simulink model "linearisedmodel"  (R2020b)
settings: Solver=VariableStepAuto  StartTime=0.0  StopTime=10.0  RelTol=1e-3
values from neighbouring files (symbols this model uses):
  b = 2.8956    [myworkspace.mat]    (also in param_uav_updated.m)
  eve = 134.75    [myworkspace.mat]    (also in param_uav_updated.m = (rho.*Va^2.*S_wing/2))
  g = 9.80665    [dyn_nlin.m]    (also in myworkspace.mat = 9.81; param_uav_updated.m; uav_eom_linear_param.m)
  P =     [myworkspace.mat]    (also in param_uav_updated.m = structure of all parameters for the Aerosonde UAV vehicle de; uav_eom_linear_param.m = param_uav_updated2(alpha))
  Va = sqrt(u^2+v^2+w^2)    [dyn_nlin.m]    (also in myworkspace.mat = 20; param_uav_updated.m = 20)
libraries: shared6dof x1, simulink x1
settings Model: Creator=Obian  LastModifiedBy=Obian

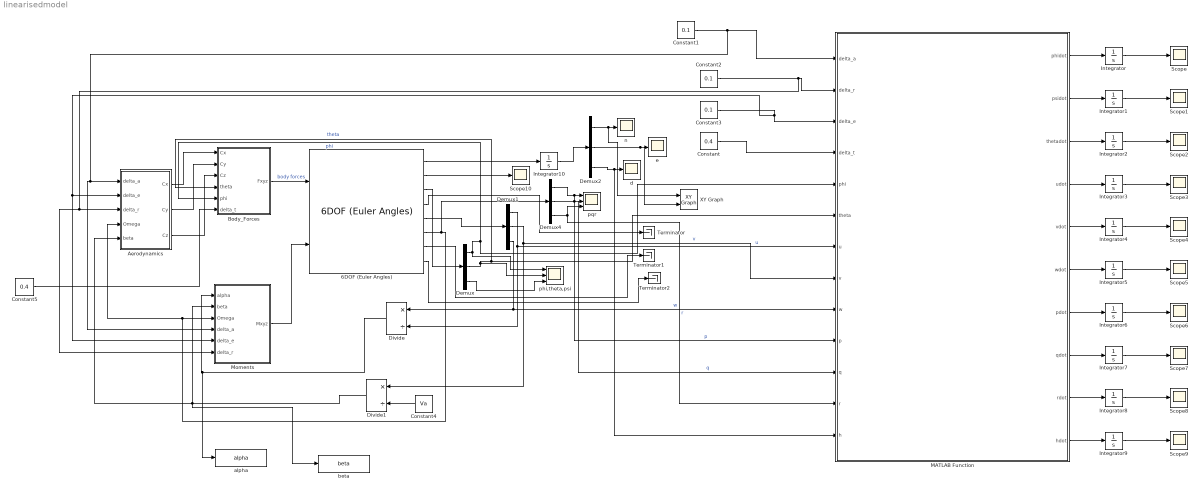
== system linearisedmodel ==
  6DOF (Euler Angles) : shared6dof/6DOF (Euler Angles)  units=Metric (MKS)  mtype=Fixed  rep=Euler Angles  xme_0=[0 0 100]  Vm_0=[20 0 0]  eul_0=[0 0 0]  pm_0=[0 0 0]  mass_0=P.mass  mass_e=0.5  mass_f=2.0  inertia=[P.Jx 0 0; 0 P.Jy 0; 0 0 P.Jz]  inertia_e=eye(3)  inertia_f=2*eye(3)  k_quat=1.0  vre_flag=on  abi_flag=off  aMode=0  xme_statename=''  Vm_statename=''  eul_statename=''  quat_statename=''  pm_statename=''  mass_statename=''
      settings: SourceProductBaseCode=AE,PW,MT,UV,VE,VP
  Aerodynamics : Subsystem
  Body_Forces : Subsystem
  Constant : Constant  Value=0.4
  Constant1 : Constant  Value=0.1
  Constant2 : Constant  Value=0.1
  Constant3 : Constant  Value=0.1
  Constant4 : Constant  Value=Va
  Constant5 : Constant  Value=0.4
  Demux{,1..2,4} (4 alike) : Demux  Outputs=3
  Divide : Product  Inputs=*/
  Divide1 : Product  Inputs=*/
  Integrator{,1..10} (11 alike) : Integrator
  MATLAB Function : MATLAB Function  TreatAsAtomicUnit=on
  Moments : Subsystem
  Scope{,1..10} (11 alike) : Scope
  Terminator : Terminator
  Terminator1 : Terminator
  Terminator2 : Terminator
  XY Graph : simulink/Sinks/XY Graph  xmin=-800  xmax=0  ymin=0  ymax=2500  st=0.01
  alpha : ToWorkspace  VariableName=alpha  SaveFormat=Timeseries  SampleTime=-1
  beta : ToWorkspace  VariableName=beta  SaveFormat=Timeseries  SampleTime=-1
  d : Scope
  e : Scope
  n : Scope
  phi,theta,psi : Scope  NumInputPorts=3
  pqr : Scope  NumInputPorts=3
  wires:
  Constant/1 -> MATLAB Function/4(delta_t)
  Integrator9/1 -> Scope9/1
  Integrator8/1 -> Scope8/1
  Integrator/1 -> Scope/1
  Integrator1/1 -> Scope1/1
  Integrator2/1 -> Scope2/1
  Integrator3/1 -> Scope3/1
  Integrator4/1 -> Scope4/1
  Integrator5/1 -> Scope5/1
  Integrator6/1 -> Scope6/1
  Integrator7/1 -> Scope7/1
  MATLAB Function/1(phidot) -> Integrator/1
  MATLAB Function/2(psidot) -> Integrator1/1
  MATLAB Function/3(thetadot) -> Integrator2/1
  MATLAB Function/4(udot) -> Integrator3/1
  MATLAB Function/5(vdot) -> Integrator4/1
  MATLAB Function/6(wdot) -> Integrator5/1
  MATLAB Function/7(pdot) -> Integrator6/1
  MATLAB Function/8(qdot) -> Integrator7/1
  MATLAB Function/9(rdot) -> Integrator8/1
  MATLAB Function/10(hdot) -> Integrator9/1
  Constant1/1 -> Moments/4(delta_a), Aerodynamics/1(delta_a), MATLAB Function/1(delta_a)
  6DOF (Euler Angles)/8 -> Terminator2/1
  6DOF (Euler Angles)/5 -> Demux1/1
  6DOF (Euler Angles)/4 -> Terminator/1
  6DOF (Euler Angles)/7 -> Terminator1/1
  6DOF (Euler Angles)/2 -> Scope10/1
  Demux4/1 -> MATLAB Function/10(p), pqr/1  "p"
  Demux4/3 -> MATLAB Function/12(r), pqr/3  "r"
  Divide1/1 -> beta/1, Moments/2(beta), Aerodynamics/5(beta)
  Constant3/1 -> Moments/5(delta_e), Aerodynamics/2(delta_e), MATLAB Function/3(delta_e)
  Integrator10/1 -> Demux2/1
  Constant5/1 -> Body_Forces/6(delta_t)
  Demux2/1 -> XY Graph/1, n/1
  6DOF (Euler Angles)/1 -> Integrator10/1
  Demux2/2 -> XY Graph/2, e/1
  Constant4/1 -> Divide1/2
  Demux2/3 -> MATLAB Function/13(h), d/1
  Divide/1 -> alpha/1, Moments/1(alpha)
  Demux/3 -> phi,theta,psi/3
  Demux1/2 -> Divide1/1, MATLAB Function/8(v)  "v"
  Demux/2 -> Body_Forces/4(theta), MATLAB Function/6(theta), phi,theta,psi/2  "theta"
  Demux/1 -> Body_Forces/5(phi), MATLAB Function/5(phi), phi,theta,psi/1  "phi"
  6DOF (Euler Angles)/3 -> Demux/1
  6DOF (Euler Angles)/6 -> Demux4/1, Aerodynamics/4(Omega), Moments/3(Omega)
  Aerodynamics/1(Cx) -> Body_Forces/1(Cx)
  Moments/1(Mxyz) -> 6DOF (Euler Angles)/2
  Body_Forces/1(Fxyz) -> 6DOF (Euler Angles)/1  "body forces"
  Demux4/2 -> MATLAB Function/11(q), pqr/2  "q"
  Aerodynamics/3(Cz) -> Body_Forces/3(Cz)
  Demux1/1 -> MATLAB Function/7(u), Divide/2  "u"
  Aerodynamics/2(Cy) -> Body_Forces/2(Cy)
  Demux1/3 -> MATLAB Function/9(w), Divide/1  "w"
  Constant2/1 -> Moments/6(delta_r), Aerodynamics/3(delta_r), MATLAB Function/2(delta_r)

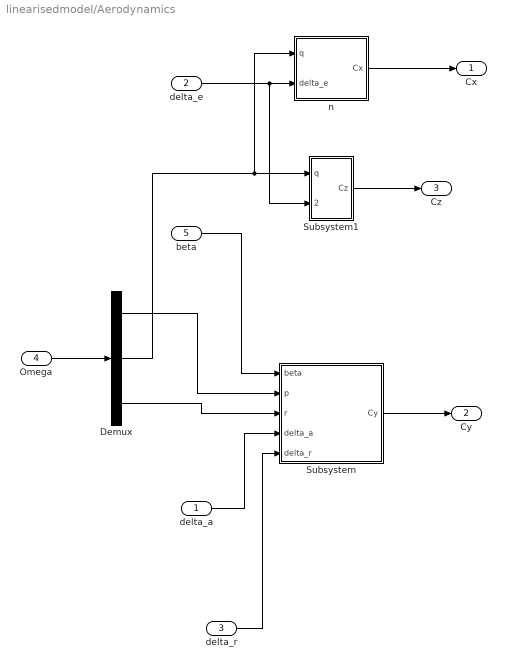
== system linearisedmodel/Aerodynamics ==
  delta_a : Inport
  delta_e : Inport  Port=2
  delta_r : Inport  Port=3
  Omega : Inport  Port=4
  beta : Inport  Port=5
  Demux : Demux  Outputs=3
  Subsystem : Subsystem
  Subsystem1 : Subsystem
  n : Subsystem
  Cx : Outport
  Cy : Outport  Port=2
  Cz : Outport  Port=3
  wires:
  Demux/2 -> n/1(q), Subsystem1/1(q)
  beta/1 -> Subsystem/1(beta)
  delta_a/1 -> Subsystem/4(delta_a)
  delta_e/1 -> Subsystem1/2(delta_e), n/2(delta_e)
  delta_r/1 -> Subsystem/5(delta_r)
  n/1(Cx) -> Cx/1
  Subsystem1/1(Cz) -> Cz/1
  Subsystem/1(Cy) -> Cy/1
  Demux/1 -> Subsystem/2(p)
  Demux/3 -> Subsystem/3(r)
  Omega/1 -> Demux/1

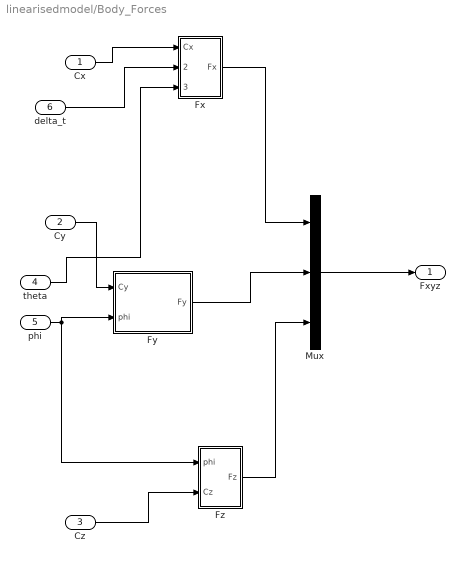
== system linearisedmodel/Body_Forces ==
  Cx : Inport
  Cy : Inport  Port=2
  Cz : Inport  Port=3
  theta : Inport  Port=4
  phi : Inport  Port=5
  delta_t : Inport  Port=6
  Fx : Subsystem
  Fy : Subsystem
  Fz : Subsystem
  Mux : Mux  Inputs=3
  Fxyz : Outport
  wires:
  Cx/1 -> Fx/1(Cx)
  Fx/1(Fx) -> Mux/1
  phi/1 -> Fz/1(phi), Fy/2(phi)
  theta/1 -> Fx/3(theta)
  Cy/1 -> Fy/1(Cy)
  Fy/1(Fy) -> Mux/2
  Fz/1(Fz) -> Mux/3
  Mux/1 -> Fxyz/1
  Cz/1 -> Fz/2(Cz)
  delta_t/1 -> Fx/2(delta_t)

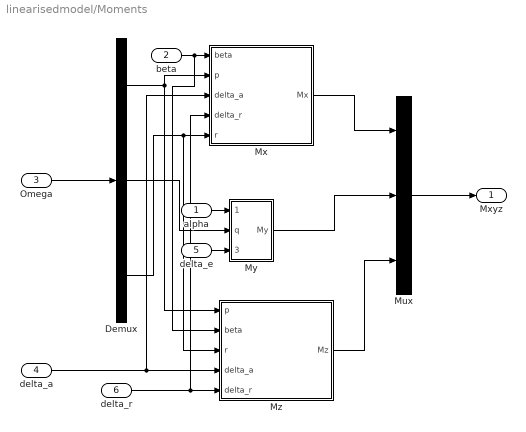
== system linearisedmodel/Moments ==
  alpha : Inport
  beta : Inport  Port=2
  Omega : Inport  Port=3
  delta_a : Inport  Port=4
  delta_e : Inport  Port=5
  delta_r : Inport  Port=6
  Demux : Demux  Outputs=3
  Mux : Mux  Inputs=3
  Mx : Subsystem
  My : Subsystem
  Mz : Subsystem
  Mxyz : Outport
  wires:
  delta_a/1 -> Mx/3(delta_a), Mz/4(delta_a)
  Mz/1(Mz) -> Mux/3
  Demux/2 -> My/2(q)
  Demux/3 -> Mz/3(r), Mx/5(r)
  Demux/1 -> Mz/1(p), Mx/2(p)
  delta_e/1 -> My/3(delta_e)
  delta_r/1 -> Mx/4(delta_r), Mz/5(delta_r)
  alpha/1 -> My/1(alpha)
  Mx/1(Mx) -> Mux/1
  Omega/1 -> Demux/1
  My/1(My) -> Mux/2
  Mux/1 -> Mxyz/1
  beta/1 -> Mz/2(beta), Mx/1(beta)

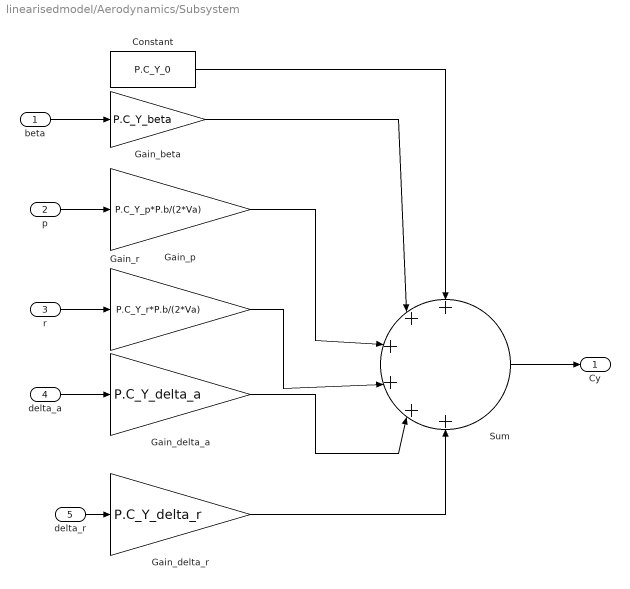
== system linearisedmodel/Aerodynamics/Subsystem ==
  beta : Inport
  p : Inport  Port=2
  r : Inport  Port=3
  delta_a : Inport  Port=4
  delta_r : Inport  Port=5
  Constant : Constant  Value=P.C_Y_0
  Gain_beta : Gain  Gain=P.C_Y_beta
  Gain_delta_a : Gain  Gain=P.C_Y_delta_a
  Gain_delta_r : Gain  Gain=P.C_Y_delta_r
  Gain_p : Gain  Gain=P.C_Y_p*P.b/(2*Va)
  Gain_r : Gain  Gain=P.C_Y_r*P.b/(2*Va)
  Sum : Sum  Inputs=++++++
  Cy : Outport
  wires:
  p/1 -> Gain_p/1
  Gain_r/1 -> Sum/4
  Gain_beta/1 -> Sum/2
  Gain_p/1 -> Sum/3
  delta_a/1 -> Gain_delta_a/1
  beta/1 -> Gain_beta/1
  Gain_delta_r/1 -> Sum/6
  Sum/1 -> Cy/1
  r/1 -> Gain_r/1
  Constant/1 -> Sum/1
  Gain_delta_a/1 -> Sum/5
  delta_r/1 -> Gain_delta_r/1

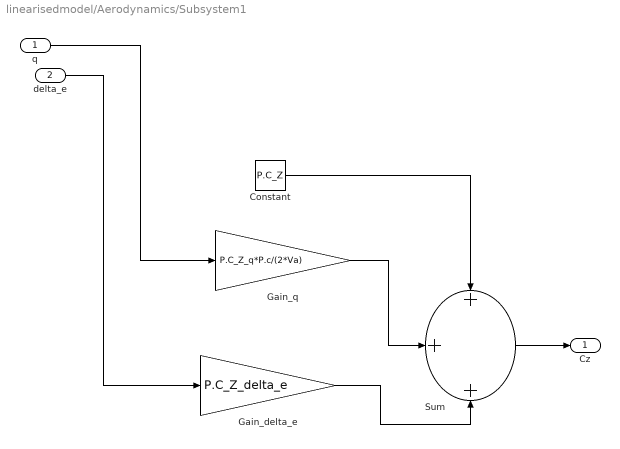
== system linearisedmodel/Aerodynamics/Subsystem1 ==
  q : Inport
  delta_e : Inport  Port=2
  Constant : Constant  Value=P.C_Z
  Gain_delta_e : Gain  Gain=P.C_Z_delta_e
  Gain_q : Gain  Gain=P.C_Z_q*P.c/(2*Va)
  Sum : Sum  Inputs=+++
  Cz : Outport
  wires:
  Sum/1 -> Cz/1
  Gain_q/1 -> Sum/2
  Gain_delta_e/1 -> Sum/3
  Constant/1 -> Sum/1
  delta_e/1 -> Gain_delta_e/1
  q/1 -> Gain_q/1

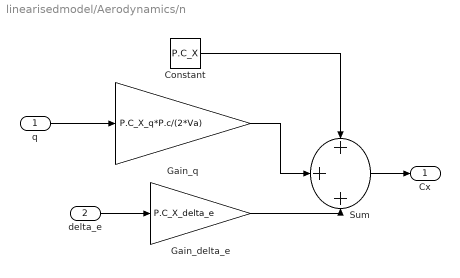
== system linearisedmodel/Aerodynamics/n ==
  q : Inport
  delta_e : Inport  Port=2
  Constant : Constant  Value=P.C_X
  Gain_delta_e : Gain  Gain=P.C_X_delta_e
  Gain_q : Gain  Gain=P.C_X_q*P.c/(2*Va)
  Sum : Sum  Inputs=+++
  Cx : Outport
  wires:
  Constant/1 -> Sum/1
  Gain_delta_e/1 -> Sum/3
  q/1 -> Gain_q/1
  Sum/1 -> Cx/1
  Gain_q/1 -> Sum/2
  delta_e/1 -> Gain_delta_e/1

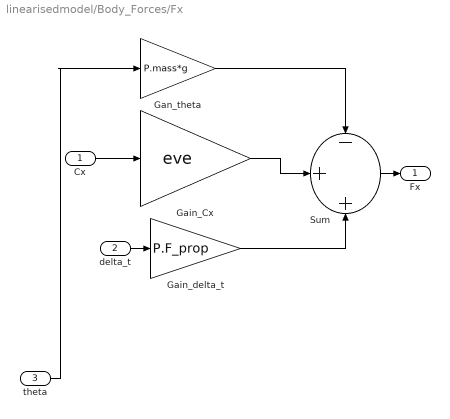
== system linearisedmodel/Body_Forces/Fx ==
  Cx : Inport
  delta_t : Inport  Port=2
  theta : Inport  Port=3
  Gain_Cx : Gain  Gain=eve
  Gain_delta_t : Gain  Gain=P.F_prop
  Gan_theta : Gain  Gain=P.mass*g
  Sum : Sum  Inputs=-++
  Fx : Outport
  wires:
  Gan_theta/1 -> Sum/1
  Gain_Cx/1 -> Sum/2
  Gain_delta_t/1 -> Sum/3
  Cx/1 -> Gain_Cx/1
  delta_t/1 -> Gain_delta_t/1
  Sum/1 -> Fx/1
  theta/1 -> Gan_theta/1

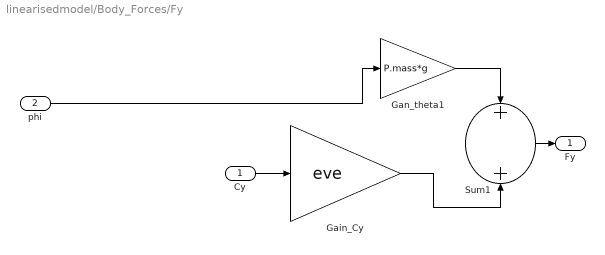
== system linearisedmodel/Body_Forces/Fy ==
  Cy : Inport
  phi : Inport  Port=2
  Gain_Cy : Gain  Gain=eve
  Gan_theta1 : Gain  Gain=P.mass*g
  Sum1 : Sum
  Fy : Outport
  wires:
  Gan_theta1/1 -> Sum1/1
  Sum1/1 -> Fy/1
  Cy/1 -> Gain_Cy/1
  Gain_Cy/1 -> Sum1/2
  phi/1 -> Gan_theta1/1

== system linearisedmodel/Body_Forces/Fz ==
  phi : Inport
  Cz : Inport  Port=2
  Gain_Cz : Gain  Gain=eve
  Gan_theta1 : Gain  Gain=P.mass*g
  Sum1 : Sum
  Fz : Outport
  wires:
  Gain_Cz/1 -> Sum1/2
  Cz/1 -> Gain_Cz/1
  Sum1/1 -> Fz/1
  Gan_theta1/1 -> Sum1/1
  phi/1 -> Gan_theta1/1

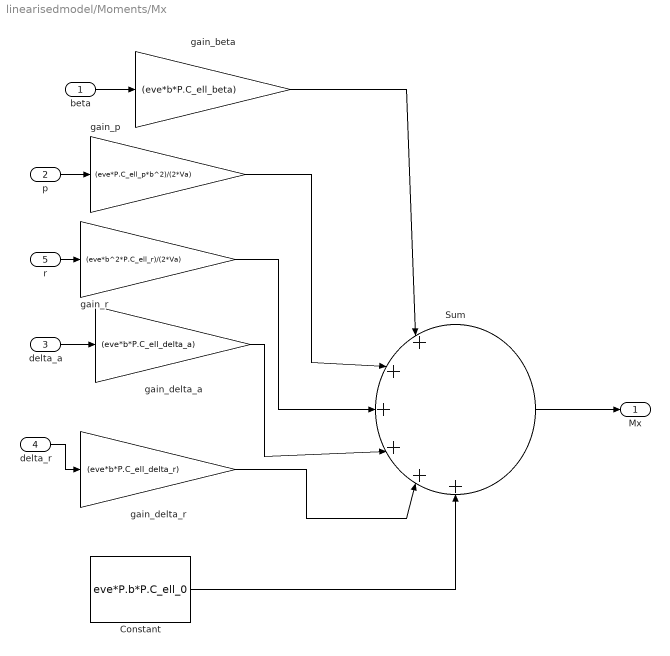
== system linearisedmodel/Moments/Mx ==
  beta : Inport
  p : Inport  Port=2
  delta_a : Inport  Port=3
  delta_r : Inport  Port=4
  r : Inport  Port=5
  Constant : Constant  Value=eve*P.b*P.C_ell_0
  Sum : Sum  Inputs=|++++++
  gain_beta : Gain  Gain=(eve*b*P.C_ell_beta)
  gain_delta_a : Gain  Gain=(eve*b*P.C_ell_delta_a)
  gain_delta_r : Gain  Gain=(eve*b*P.C_ell_delta_r)
  gain_p : Gain  Gain=(eve*P.C_ell_p*b^2)/(2*Va)
  gain_r : Gain  Gain=(eve*b^2*P.C_ell_r)/(2*Va)
  Mx : Outport
  wires:
  gain_beta/1 -> Sum/1
  delta_r/1 -> gain_delta_r/1
  p/1 -> gain_p/1
  r/1 -> gain_r/1
  gain_p/1 -> Sum/2
  delta_a/1 -> gain_delta_a/1
  gain_r/1 -> Sum/3
  beta/1 -> gain_beta/1
  gain_delta_r/1 -> Sum/5
  Sum/1 -> Mx/1
  Constant/1 -> Sum/6
  gain_delta_a/1 -> Sum/4

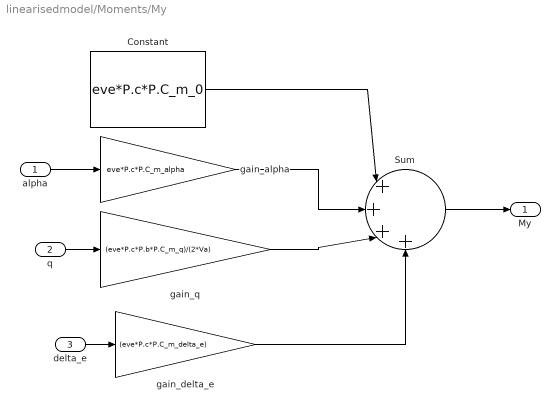
== system linearisedmodel/Moments/My ==
  alpha : Inport
  q : Inport  Port=2
  delta_e : Inport  Port=3
  Constant : Constant  Value=eve*P.c*P.C_m_0
  Sum : Sum  Inputs=|++++
  gain_alpha : Gain  Gain=eve*P.c*P.C_m_alpha
  gain_delta_e : Gain  Gain=(eve*P.c*P.C_m_delta_e)
  gain_q : Gain  Gain=(eve*P.c*P.b*P.C_m_q)/(2*Va)
  My : Outport
  wires:
  Sum/1 -> My/1
  gain_delta_e/1 -> Sum/4
  gain_q/1 -> Sum/3
  q/1 -> gain_q/1
  delta_e/1 -> gain_delta_e/1
  gain_alpha/1 -> Sum/2
  Constant/1 -> Sum/1
  alpha/1 -> gain_alpha/1

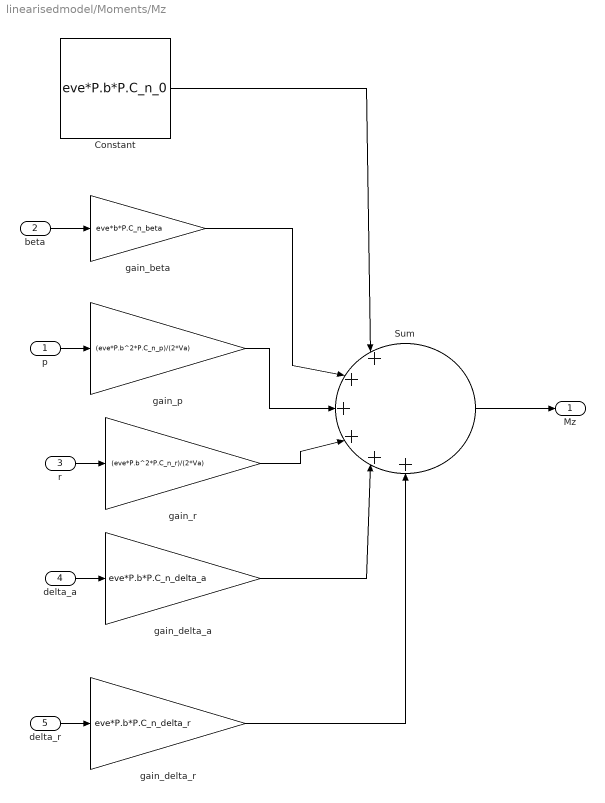
== system linearisedmodel/Moments/Mz ==
  p : Inport
  beta : Inport  Port=2
  r : Inport  Port=3
  delta_a : Inport  Port=4
  delta_r : Inport  Port=5
  Constant : Constant  Value=eve*P.b*P.C_n_0
  Sum : Sum  Inputs=|++++++
  gain_beta : Gain  Gain=eve*b*P.C_n_beta
  gain_delta_a : Gain  Gain=eve*P.b*P.C_n_delta_a
  gain_delta_r : Gain  Gain=eve*P.b*P.C_n_delta_r
  gain_p : Gain  Gain=(eve*P.b^2*P.C_n_p)/(2*Va)
  gain_r : Gain  Gain=(eve*P.b^2*P.C_n_r)/(2*Va)
  Mz : Outport
  wires:
  p/1 -> gain_p/1
  beta/1 -> gain_beta/1
  gain_delta_r/1 -> Sum/6
  delta_a/1 -> gain_delta_a/1
  gain_r/1 -> Sum/4
  Constant/1 -> Sum/1
  gain_p/1 -> Sum/3
  Sum/1 -> Mz/1
  gain_delta_a/1 -> Sum/5
  gain_beta/1 -> Sum/2
  delta_r/1 -> gain_delta_r/1
  r/1 -> gain_r/1

== matlab function linearisedmodel/MATLAB Function ==
  data: delta_a input; delta_r input; delta_e input; delta_t input; phidot output; psidot output; thetadot output; phi input; theta input; u input; v input; w input; p input; q input; r input; h input; udot output; vdot output; wdot output; pdot output; qdot output; rdot output; hdot output
function [phidot, psidot, thetadot, udot, vdot, wdot, pdot, qdot, rdot, hdot] = fcn(delta_a, delta_r, delta_e, delta_t, phi, theta, u, v, w, p, q, r, h)

P = uav1(alpha);

Va = 27.3; %airspeed, m/s

% constants
g = 9.80665; % gravitational acceleration, P.mass/s^2
rho =  1.2133;  %kg/P.mass^3, density of air at 100 P.mass height (assume to be constant)
% alpha=0;

beta = 0.1;

psi=0;



%% LATERAL state-space, x = [v p r phi, psi]
Yv = (rho*P.S_wing*P.b*v/(4*P.mass*Va))*(P.C_Y_p*p + P.C_Y_r*r) ...
    + (rho*P.S_wing*v/P.mass)*(P.C_Y_0+P.C_Y_beta+P.C_Y_delta_a*delta_a+P.C_Y_delta_r*delta_r)...
    + (rho*P.S_wing*P.C_Y_beta/(2*P.mass))*norm([u, w]);
Yp = w + (rho*Va*P.S_wing*P.b/(4*P.mass))*P.C_Y_p;
Yr = -u + (rho*Va*P.S_wing*P.b/(4*P.mass))*P.C_Y_r;
Yda = (rho*Va^2*P.S_wing/(2*P.mass))*P.C_Y_delta_a;
Ydr = (rho*Va^2*P.S_wing/(2*P.mass))*P.C_Y_delta_r;

Lv = (rho*P.S_wing*P.b^2*v/(4*Va))*(P.C_p_p*p + P.C_p_r*r) ...
    + (rho*P.S_wing*P.b*v)*(P.C_p_0+P.C_p_beta+P.C_p_delta_a*delta_a+P.C_p_delta_r*delta_r)...
    + (rho*P.S_wing*P.b*P.C_p_beta/2)*norm([u, w]);
Lp = P.Gamma_1*q + (rho*Va*P.S_wing*P.b^2/4)*P.C_p_p;
Lr = -P.Gamma_2*q + (rho*Va*P.S_wing*P.b^2/4)*P.C_p_r;
Lda = (rho*Va^2*P.S_wing*P.b/2)*P.C_p_delta_a;
Ldr = (rho*Va^2*P.S_wing*P.b/2)*P.C_p_delta_r;

Nv = (rho*P.S_wing*P.b^2*v/(4*Va))*(P.C_r_p*p + P.C_r_r*r) ...
    + (rho*P.S_wing*P.b*v)*(P.C_r_0+P.C_r_beta+P.C_r_delta_a*delta_a+P.C_r_delta_r*delta_r)...
    + (rho*P.S_wing*P.b*P.C_r_beta)*norm([u, w]);
Np = P.Gamma_7*q + (rho*Va*P.S_wing*P.b^2/4)*P.C_r_p;
Nr = -P.Gamma_1*q + (rho*Va*P.S_wing*P.b^2/4)*P.C_r_r;
Nda = (rho*Va^2*P.S_wing*P.b/2)*P.C_r_delta_a;
Ndr = (rho*Va^2*P.S_wing*P.b/2)*P.C_r_delta_r;

%% LONGITUDINAL state space, x = [u w q theta h]
Xu = (u*rho*P.S_wing/P.mass)*(P.C_X_0+P.C_X_alpha+P.C_X_delta_e*delta_e) - (rho*P.S_wing*w*P.C_X_alpha/(2*P.mass)) ...
    + (rho*P.S_wing*P.c*P.C_X_q*u*q/(4*P.mass*Va)); %- (rho*Sprop*Cprop*u/P.mass); 
Xw = -q +  (w*rho*P.S_wing/P.mass)*(P.C_X_0+P.C_X_alpha+P.C_X_delta_e*delta_e) + (rho*P.S_wing*u*P.C_X_alpha/(2*P.mass)) ...
    + (rho*P.S_wing*P.c*P.C_X_q*w*q/(4*P.mass*Va)); %(rho*Sprop*Cprop*w/P.mass); 
Xq = -w + (rho*Va*P.S_wing*P.C_X_q*P.c)/(4*P.mass);
Xde = (rho*Va^2*P.S_wing*P.C_X_delta_e)/(2*P.mass);
% Xdt = rho*Sprop*Cprop*k^2*delta_t/P.mass;
Xdt = P.F_prop/P.mass;

Zu = q +  (u*rho*P.S_wing/P.mass)*(P.C_Z_0+P.C_Z_alpha+P.C_Z_delta_e*delta_e) - (rho*P.S_wing*w*P.C_Z_alpha/(2*P.mass)) ...
    + (u*rho*P.S_wing*P.c*P.C_Z_q*q/(4*P.mass*Va));  
Zw = (w*rho*P.S_wing/P.mass)*(P.C_Z_0+P.C_Z_alpha+P.C_Z_delta_e*delta_e) + (rho*P.S_wing*u*P.C_Z_alpha/(2*P.mass)) ...
    + (w*rho*P.S_wing*P.c*P.C_Z_q*q/(4*P.mass*Va));  
Zq = u + (rho*Va*P.S_wing*P.C_X_q*P.c)/(4*P.mass);
Zde = (rho*Va^2*P.S_wing*P.C_X_delta_e)/(2*P.mass);

Mu = (u*rho*P.S_wing*P.c/P.Jy)*(P.C_m_0+P.C_m_alpha+P.C_m_delta_e*delta_e) - (rho*P.S_wing*P.c*P.C_m_alpha*w)/(2*P.Jy) ...
    + (rho*P.S_wing*P.c^2*P.C_m_q*q*u)/(4*P.Jy*Va);
Mw = (w*rho*P.S_wing*P.c/P.Jy)*(P.C_m_0+P.C_m_alpha+P.C_m_delta_e*delta_e) + (rho*P.S_wing*P.c*P.C_m_alpha*u)/(2*P.Jy) ...
    + (rho*P.S_wing*P.c^2*P.C_m_q*q*w)/(4*P.Jy*Va);
Mq = (rho*Va*P.S_wing*P.c^2*P.C_m_q)/(4*P.Jy);
Mde = (rho*Va^2*P.S_wing*P.c*P.C_m_delta_e)/(4*P.Jy);

theta_star = theta - 0.60269;
phi_star = phi - 1.161;
% q_star = q;
% p_star = p;
% r = r;
u_star = u - 22.4175;
w_star = w - 3.7501;

        % Lateral space model
        
        vdot=Yv*v+Yp*p+Yr*r+g*cos(theta_star)*cos(phi_star)*phi+Yda*delta_a+Ydr*delta_r;
        pdot=Lv*v+Lp*p+Lr*r+Lda*delta_a+Ldr*delta_r;
        rdot=Nv*v+Np*p+Nr*r+Nda*delta_a+Ndr*delta_r;
        phidot=p+cos(phi_star)*tan(theta_star)*r*sin(phi_star)*tan(theta_star);
        psidot=cos(phi_star)*sec(theta_star)*r+p*cos(phi_star)*sec(theta_star)*phi;

   

        % Longitudinal space model

        udot = Xu*u + Xw*w + Xq*q -g*cos(theta_star)*theta + Xde*delta_e + Xdt*delta_t;
        wdot = Zu*u + Zw*w + Zq*q -g*sin(theta_star)*theta + Zde*delta_e;
        qdot = Mu*u + Mw*w + Mq*q + Mde*delta_e;
        thetadot = q;
        hdot = sin(theta_star)*u -cos(theta_star)*w + (u_star*cos(theta_star)+w_star*sin(theta_star))*theta;
        
%         % n, e, h from euler transformation
%         ndot = u*cos(theta)*cos(psi) + v*(sin(phi)*sin(theta)*cos(psi) - cos(phi)*sin(psi)) + w*(cos(phi)*sin(theta)*cos(psi) + sin(phi)*sin(psi));
%         edot = u*cos(theta)*sin(psi) + v*(sin(phi)*sin(theta)*sin(psi) + cos(phi)*cos(psi)) + w*(cos(phi)*sin(theta)*sin(psi) - sin(phi)*cos(psi));
%         hdot = -u*sin(theta) + v*sin(phi)*cos(theta) + w*cos(phi)*cos(theta);  % h = -pz

return
